simulink model "WK_MaoBi_circle_25102013_Offline"  (Simulink 7.7)
settings: Solver=ode4  StartTime=0.0  StopTime=inf  FixedStep=sample_time  RelTol=1e-3
InitFcn:
  | sample_time=0.005;%0.004;%0.0025;%0.02;
  | DeltaT = 0.02;
  | g = 9.81;
  | H0 = g%0.3165;
  | Kl = 1;
  | 
  | Omega_r = 1.6;%for Horizontal reference
  | Zeta_r = 0.7; %for Horizontal reference
  | Omega = 1.8;%for Horizontal Control
  | Zeta = 0.5;    %for Horizontal Control
  | 
  | Omega_h_r = 2.5; %for vertical reference
  | Zeta_h_r = 0.8;  %for vertical reference
  | Omega_h = 2.7;    %for vertical control
  | Zeta_h = 0.8;         %for vertical control
  | PI=pi;
  | 
  | Mass = 1.1;
  | Acc_Max = 4;
  | Acc_Max_h = 4;
  | 
  | Max_RP = 60;
  | 
  | load MaoBi_Oct04_2_int.mat
  | MB_Interp.time = [];
undefined symbols (not defined in the file or in its folder): DiscIntNeverNeededParam
libraries: simulink x7, dspadpt3 x3, X330_Control x2, X400_Control x1
(part 2 of 2)

== stateflow chart Planning/Trajectory Logic/UAV SF ==
  state Landing
    state Descending
      en:PosDesired = Pos;
      du:PosDesired[2] = (PerchPos[2]- PosDesired[2])*1*DeltaT + PosDesired[2] ;
    state CutThrottle
      du:HoverThrottle = (0 - HoverThrottle)*3*DeltaT + HoverThrottle ;
    (default) -> Descending
    Descending -> CutThrottle : [Pos[2] > (PerchPos[2]-0.1)]
  state Airborne
    state TakeOff
      du:HoverThrottle = (H0 - HoverThrottle)*3*DeltaT + HoverThrottle ;
    state Descent1
      descentrate=descentrate+0.01;
    state Descent
      en:PosDesired[2] = PerchPos[2]-0.2+descentrate;
    state SafyHover
      en:PosDesired = Pos; PosDesired[2]=-1.2;
    state Prelanding
      en:PosDesired[0] = PerchPos[0]; PosDesired[1] = PerchPos[1];PosDesired[2] = PerchPos[2]-0.5 ;
      descentrate=0;
    state Loop
      state drawing_circle_line
        en:
        PosDesired[0]=draw[0]+xoffset-0.25, PosDesired[1]=draw[1],PosDesired[2]= draw[2]-Heightcontrol-0.1;
      state MBdown
        en:
        PosDesired[0]=draw[0]+xoffset-0.25+0.1cos(degree);
        PosDesired[1]=draw[1]+0.1sin(degree);
        PosDesired[2]=draw[2]-Heightcontrol;
      state End_Point
        en:
        PosDesired[0]=draw[0]+xoffset-0.25, PosDesired[1]=draw[1]+0.1,PosDesired[2]= draw[2]-Heightcontrol;
      state MBup
        en:
        PosDesired[2]= draw[2]-Heightcontrol-0.1;
      state drawing_circle_line1
        en:
        degree=degree+changeindegree;
        PosDesired[2]=draw[2]-Heightcontrol;
      drawing_circle_line -> MBdown : [abs(PosDesired[0]-draw[0]+xoffset-0.25)+abs(PosDesired[1]-draw[1])<0.1]
      MBdown -> drawing_circle_line1 [order 1] : [degree<180]
      End_Point -> MBup : after (1,sec)
      MBdown -> End_Point [order 2] : [abs(PosDesired[1]-draw[1]-0.1)<0.01]
      drawing_circle_line1 -> MBdown : after(2,sec)
      (default) -> drawing_circle_line
    state TakeOff1
      count=0;
    Loop -> SafyHover : [RC[5] > 0]
    (default) -> TakeOff : {PosDesired = Pos;  PosDesired[2] =-1.2;}
    TakeOff -> TakeOff1 [order 1] : after(5,sec)
    SafyHover -> Prelanding : after (3, sec)
    Prelanding -> Descent : [PerchError < 0.01]
    Descent -> Descent1 [order 2] : [PerchError < 0.01]
    TakeOff1 -> Loop
    Descent -> Prelanding [order 1] : after (5,sec)
    Descent1 -> Descent : after (0.5,sec)
    TakeOff -> SafyHover [order 2] : [RC[5] > 0]
  (default) -> Landing : {HoverThrottle = 0;}
  Airborne -> Landing : [RC[6] < -0.5]
  Landing -> Airborne : [RC[6] > 0.5]
  data: PosDesired output double size=4; HoverThrottle output double size=1; Mode output uint8 size=1; RC input double size=8; Pos input double size=4; PerchPos input double size=4; DeltaT parameter double size=1; H0 parameter double size=1; Kl parameter double size=1; VelCmd local double size=2 =0; PWM output double; PerchError input double; PI parameter double size=1; draw input double size=3; Heightcontrol input double; degree input double; xoffset input double; descentrate local double; changeindegree input double
